simulink model "SMC_01"  (R2021a)
settings: Solver=ode14x  StartTime=0.0  StopTime=30  FixedStep=0.01  RelTol=1e-3
libraries: simulink x2
settings Model: Creator=TMP  LastModifiedBy=TMP

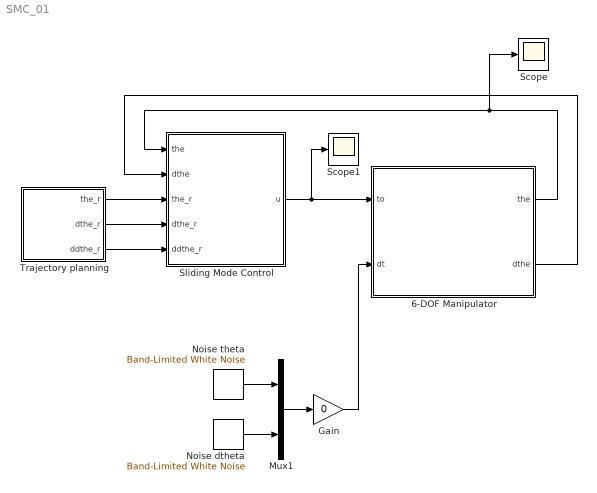
== system SMC_01 ==
  6-DOF Manipulator : Subsystem
  Gain : Gain  Gain=0
  Mux1 : Mux  Inputs=2
  Noise dtheta : simulink/Sources/Band-Limited White Noise  Cov=[0.03]  Ts=0.01  seed=[23341]
  Noise theta : simulink/Sources/Band-Limited White Noise  Cov=[0.003]  Ts=0.01  seed=[23341]
  Scope : Scope
  Scope1 : Scope
  Sliding Mode Control : MATLAB Function  TreatAsAtomicUnit=on
  Trajectory planning : Subsystem
  wires:
  Sliding Mode Control/1(u) -> Scope1/1, 6-DOF Manipulator/1(to)
  Noise theta/1 -> Mux1/1
  Noise dtheta/1 -> Mux1/2
  Gain/1 -> 6-DOF Manipulator/2(dt)
  Mux1/1 -> Gain/1
  6-DOF Manipulator/2(dthe) -> Sliding Mode Control/2(dthe)
  6-DOF Manipulator/1(the) -> Scope/1, Sliding Mode Control/1(the)
  Trajectory planning/3(ddthe_r) -> Sliding Mode Control/5(ddthe_r)
  Trajectory planning/2(dthe_r) -> Sliding Mode Control/4(dthe_r)
  Trajectory planning/1(the_r) -> Sliding Mode Control/3(the_r)

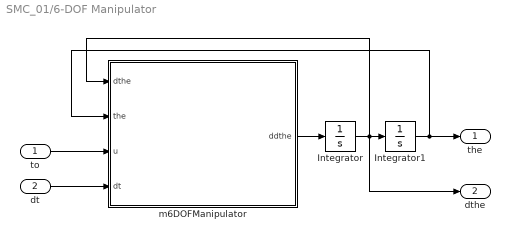
== system SMC_01/6-DOF Manipulator ==
  to : Inport
  dt : Inport  Port=2
  Integrator : Integrator  InitialCondition=[0.01;0.01;0.01;0.01;0.01;0.01]
  Integrator1 : Integrator  InitialCondition=[0.01;0.01;0.01;0.01;0.01;0.01]
  m6DOFManipulator : MATLAB Function  TreatAsAtomicUnit=on
  the : Outport
  dthe : Outport  Port=2
  wires:
  Integrator1/1 -> the/1, m6DOFManipulator/2(the)
  m6DOFManipulator/1(ddthe) -> Integrator/1
  Integrator/1 -> dthe/1, m6DOFManipulator/1(dthe), Integrator1/1
  dt/1 -> m6DOFManipulator/4(dt)
  to/1 -> m6DOFManipulator/3(u)

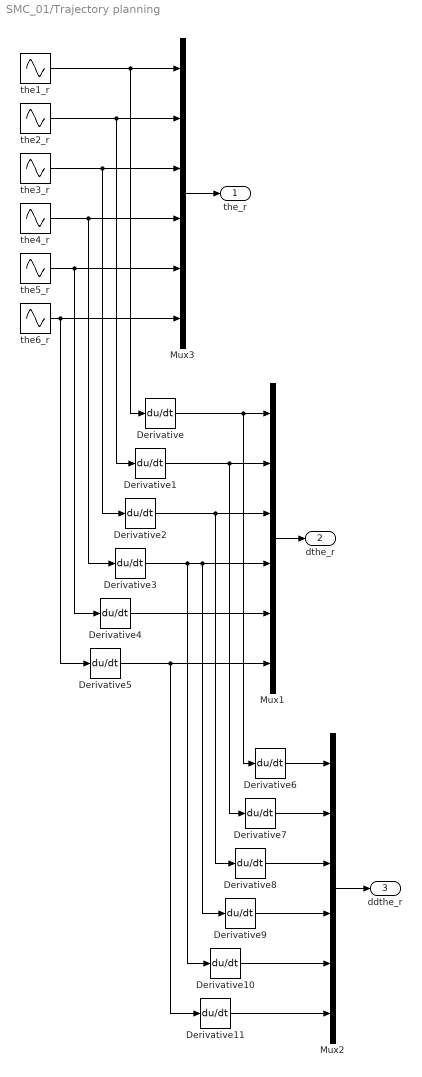
== system SMC_01/Trajectory planning ==
  Derivative{,1..11} (12 alike) : Derivative
  Mux1 : Mux  Inputs=6
  Mux2 : Mux  Inputs=6
  Mux3 : Mux  Inputs=6
  the1_r : Sin  Amplitude=pi/3  Frequency=2*pi*0.1  SampleTime=0
  the2_r : Sin  Amplitude=pi/4  Frequency=2*pi*0.1  SampleTime=0
  the3_r : Sin  Amplitude=pi/6  Frequency=2*pi*0.1  SampleTime=0
  the4_r : Sin  Amplitude=pi/3  Frequency=2*pi*0.1  Phase=pi/3  SampleTime=0
  the5_r : Sin  Amplitude=pi/4  Frequency=2*pi*0.1  Phase=pi/4  SampleTime=0
  the6_r : Sin  Amplitude=pi/6  Frequency=2*pi*0.1  Phase=pi/6  SampleTime=0
  the_r : Outport  VectorParamsAs1DForOutWhenUnconnected=off
  dthe_r : Outport  Port=2  VectorParamsAs1DForOutWhenUnconnected=off
  ddthe_r : Outport  Port=3  VectorParamsAs1DForOutWhenUnconnected=off
  wires:
  the1_r/1 -> Derivative/1, Mux3/1
  the2_r/1 -> Derivative1/1, Mux3/2
  the3_r/1 -> Derivative2/1, Mux3/3
  the4_r/1 -> Derivative3/1, Mux3/4
  the5_r/1 -> Derivative4/1, Mux3/5
  the6_r/1 -> Derivative5/1, Mux3/6
  Derivative/1 -> Derivative6/1, Mux1/1
  Derivative1/1 -> Derivative7/1, Mux1/2
  Derivative2/1 -> Derivative8/1, Mux1/3
  Derivative3/1 -> Derivative10/1, Derivative9/1, Mux1/4
  Derivative4/1 -> Mux1/5
  Derivative5/1 -> Derivative11/1, Mux1/6
  Mux3/1 -> the_r/1
  Derivative6/1 -> Mux2/1
  Derivative7/1 -> Mux2/2
  Derivative8/1 -> Mux2/3
  Derivative9/1 -> Mux2/4
  Derivative10/1 -> Mux2/5
  Derivative11/1 -> Mux2/6
  Mux1/1 -> dthe_r/1
  Mux2/1 -> ddthe_r/1

== matlab function SMC_01/Sliding Mode Control ==
  data: the input; u output; dthe input; the_r input; dthe_r input; ddthe_r input
function u = SMC(the,dthe,the_r,dthe_r,ddthe_r)
%% Declare manipulator dynamics:
m1=0.1; m2=0.1; m3=0.1; m4=0.1; m5=0.1; m6=0.1;
I1=0; I2=0; I3=0; I4=0; I5=0; I6=1;
a1=0.75; a2=2.70; a3=0.90; d1=3.35; d4=2.95; d7=0.80;
g=9.81;
%%
e1 = the(1); e2 = the(2); e3 = the(3);
e4 = the(4); e5 = the(5); e6 = the(6);
de1 = dthe(1); de2 = dthe(2); de3 = dthe(3);
de4 = dthe(4); de5 = dthe(5); de6 = dthe(6);
%% M
M = [I1 + I2 + I3 + I4 + I5 + I6 + a1^2*m2 + a1^2*m3 + a1^2*m4 + (a2^2*m3)/2 + a1^2*m5 + (a2^2*m4)/2 + a1^2*m6 + (a2^2*m5)/2 + (a3^2*m4)/2 + (a2^2*m6)/2 + (a3^2*m5)/2 + (a3^2*m6)/2 + (d4^2*m4)/2 + (d4^2*m5)/2 + (d4^2*m6)/2 - (a2^2*m3*cos(2*e2))/2 - (a2^2*m4*cos(2*e2))/2 - (a2^2*m5*cos(2*e2))/2 - (a2^2*m6*cos(2*e2))/2 - (a3^2*m4*cos(2*e2 + 2*e3))/2 - (a3^2*m5*cos(2*e2 + 2*e3))/2 - (a3^2*m6*cos(2*e2 + 2*e3))/2 + (d4^2*m4*cos(2*e2 + 2*e3))/2 + (d4^2*m5*cos(2*e2 + 2*e3))/2 + (d4^2*m6*cos(2*e2 + 2*e3))/2 + 2*a1*d4*m4*cos(e2 + e3) + 2*a1*d4*m5*cos(e2 + e3) + 2*a1*d4*m6*cos(e2 + e3) + 2*a1*a3*m4*sin(e2 + e3) + 2*a1*a3*m5*sin(e2 + e3) + 2*a1*a3*m6*sin(e2 + e3) + a2*a3*m4*cos(e3) + a2*a3*m5*cos(e3) + a2*a3*m6*cos(e3) + 2*a1*a2*m3*sin(e2) + 2*a1*a2*m4*sin(e2) + 2*a1*a2*m5*sin(e2) + 2*a1*a2*m6*sin(e2) - a2*d4*m4*sin(e3) - a2*d4*m5*sin(e3) - a2*d4*m6*sin(e3) - a2*a3*m4*cos(2*e2 + e3) - a2*a3*m5*cos(2*e2 + e3) - a2*a3*m6*cos(2*e2 + e3) + a2*d4*m4*sin(2*e2 + e3) + a2*d4*m5*sin(2*e2 + e3) + a2*d4*m6*sin(2*e2 + e3) + a3*d4*m4*sin(2*e2 + 2*e3) + a3*d4*m5*sin(2*e2 + 2*e3) + a3*d4*m6*sin(2*e2 + 2*e3),0,0,-sin(e2 + e3)*(I4 + I5 + I6),cos(e2 + e3)*sin(e4)*(I5 + I6),I6*cos(e4)*sin(e2)*sin(e3)*sin(e5) - I6*cos(e3)*cos(e5)*sin(e2) - I6*cos(e2)*cos(e3)*cos(e4)*sin(e5) - I6*cos(e2)*cos(e5)*sin(e3);
     0,I2 + I3 + I4 + I5 + I6 + a2^2*m3 + a2^2*m4 + a2^2*m5 + a3^2*m4 + a2^2*m6 + a3^2*m5 + a3^2*m6 + d4^2*m4 + d4^2*m5 + d4^2*m6 + 2*a2*a3*m4*cos(e3) + 2*a2*a3*m5*cos(e3) + 2*a2*a3*m6*cos(e3) - 2*a2*d4*m4*sin(e3) - 2*a2*d4*m5*sin(e3) - 2*a2*d4*m6*sin(e3),I3 + I4 + I5 + I6 + a3^2*m4 + a3^2*m5 + a3^2*m6 + d4^2*m4 + d4^2*m5 + d4^2*m6 + a2*a3*m4*cos(e3) + a2*a3*m5*cos(e3) + a2*a3*m6*cos(e3) - a2*d4*m4*sin(e3) - a2*d4*m5*sin(e3) - a2*d4*m6*sin(e3),0,cos(e4)*(I5 + I6),I6*sin(e4)*sin(e5);
     0,I3 + I4 + I5 + I6 + a3^2*m4 + a3^2*m5 + a3^2*m6 + d4^2*m4 + d4^2*m5 + d4^2*m6 + a2*a3*m4*cos(e3) + a2*a3*m5*cos(e3) + a2*a3*m6*cos(e3) - a2*d4*m4*sin(e3) - a2*d4*m5*sin(e3) - a2*d4*m6*sin(e3),I3 + I4 + I5 + I6 + a3^2*m4 + a3^2*m5 + a3^2*m6 + d4^2*m4 + d4^2*m5 + d4^2*m6,0,cos(e4)*(I5 + I6),I6*sin(e4)*sin(e5);
    -sin(e2 + e3)*(I4 + I5 + I6),0,0,I4 + I5 + I6,0,I6*cos(e5);
    cos(e2 + e3)*sin(e4)*(I5 + I6),cos(e4)*(I5 + I6),cos(e4)*(I5 + I6),0,I5 + I6,0;
    I6*cos(e4)*sin(e2)*sin(e3)*sin(e5) - I6*cos(e3)*cos(e5)*sin(e2) - I6*cos(e2)*cos(e3)*cos(e4)*sin(e5) - I6*cos(e2)*cos(e5)*sin(e3),I6*sin(e4)*sin(e5),I6*sin(e4)*sin(e5),I6*cos(e5),0,I6];
%% C
C = ...
[de2*(a2^2*m3*sin(2*e2) + a2^2*m4*sin(2*e2) + a2^2*m5*sin(2*e2) + a2^2*m6*sin(2*e2) + a3^2*m4*sin(2*e2 + 2*e3) + a3^2*m5*sin(2*e2 + 2*e3) + a3^2*m6*sin(2*e2 + 2*e3) - d4^2*m4*sin(2*e2 + 2*e3) - d4^2*m5*sin(2*e2 + 2*e3) - d4^2*m6*sin(2*e2 + 2*e3) + 2*a1*a3*m4*cos(e2 + e3) + 2*a1*a3*m5*cos(e2 + e3) + 2*a1*a3*m6*cos(e2 + e3) - 2*a1*d4*m4*sin(e2 + e3) - 2*a1*d4*m5*sin(e2 + e3) - 2*a1*d4*m6*sin(e2 + e3) + 2*a1*a2*m3*cos(e2) + 2*a1*a2*m4*cos(e2) + 2*a1*a2*m5*cos(e2) + 2*a1*a2*m6*cos(e2) + 2*a2*d4*m4*cos(2*e2 + e3) + 2*a2*d4*m5*cos(2*e2 + e3) + 2*a2*d4*m6*cos(2*e2 + e3) + 2*a2*a3*m4*sin(2*e2 + e3) + 2*a2*a3*m5*sin(2*e2 + e3) + 2*a2*a3*m6*sin(2*e2 + e3) + 2*a3*d4*m4*cos(2*e2 + 2*e3) + 2*a3*d4*m5*cos(2*e2 + 2*e3) + 2*a3*d4*m6*cos(2*e2 + 2*e3)) + de3*(m4 + m5 + m6)*(a3^2*sin(2*e2 + 2*e3) - d4^2*sin(2*e2 + 2*e3) + a2*d4*cos(2*e2 + e3) + a2*a3*sin(2*e2 + e3) + 2*a3*d4*cos(2*e2 + 2*e3) + 2*a1*a3*cos(e2 + e3) - 2*a1*d4*sin(e2 + e3) - a2*d4*cos(e3) - a2*a3*sin(e3)),0,0,-cos(e2 + e3)*(de2 + de3)*(I4 + I5 + I6),-(I5 + I6)*(de2*sin(e2 + e3)*sin(e4) - de4*cos(e2 + e3)*cos(e4) + de3*sin(e2 + e3)*sin(e4)),I6*de2*(cos(e5)*sin(e2)*sin(e3) - cos(e2)*cos(e3)*cos(e5) + cos(e2)*cos(e4)*sin(e3)*sin(e5) + cos(e3)*cos(e4)*sin(e2)*sin(e5)) + I6*de3*(cos(e5)*sin(e2)*sin(e3) - cos(e2)*cos(e3)*cos(e5) + cos(e2)*cos(e4)*sin(e3)*sin(e5) + cos(e3)*cos(e4)*sin(e2)*sin(e5)) + I6*de5*(cos(e2)*sin(e3)*sin(e5) + cos(e3)*sin(e2)*sin(e5) - cos(e2)*cos(e3)*cos(e4)*cos(e5) + cos(e4)*cos(e5)*sin(e2)*sin(e3)) + I6*de4*cos(e2 + e3)*sin(e4)*sin(e5);
 (I4*de4*cos(e2 + e3))/2 + (I5*de4*cos(e2 + e3))/2 + (I6*de4*cos(e2 + e3))/2 - (a2^2*de1*m3*sin(2*e2))/2 - (a2^2*de1*m4*sin(2*e2))/2 - (a2^2*de1*m5*sin(2*e2))/2 - (a2^2*de1*m6*sin(2*e2))/2 - (a3^2*de1*m4*sin(2*e2 + 2*e3))/2 - (a3^2*de1*m5*sin(2*e2 + 2*e3))/2 - (a3^2*de1*m6*sin(2*e2 + 2*e3))/2 + (d4^2*de1*m4*sin(2*e2 + 2*e3))/2 + (d4^2*de1*m5*sin(2*e2 + 2*e3))/2 + (d4^2*de1*m6*sin(2*e2 + 2*e3))/2 + (I5*de5*sin(e2 + e3)*sin(e4))/2 + (I6*de5*sin(e2 + e3)*sin(e4))/2 - a3*d4*de1*m4*cos(2*e2 + 2*e3) - a3*d4*de1*m5*cos(2*e2 + 2*e3) - a3*d4*de1*m6*cos(2*e2 + 2*e3) + (I6*de6*cos(e2)*cos(e3)*cos(e5))/2 - a1*a3*de1*m4*cos(e2 + e3) - a1*a3*de1*m5*cos(e2 + e3) - a1*a3*de1*m6*cos(e2 + e3) - (I6*de6*cos(e5)*sin(e2)*sin(e3))/2 + a1*d4*de1*m4*sin(e2 + e3) + a1*d4*de1*m5*sin(e2 + e3) + a1*d4*de1*m6*sin(e2 + e3) - a1*a2*de1*m3*cos(e2) - a1*a2*de1*m4*cos(e2) - a1*a2*de1*m5*cos(e2) - a1*a2*de1*m6*cos(e2) - a2*d4*de1*m4*cos(2*e2 + e3) - a2*d4*de1*m5*cos(2*e2 + e3) - a2*d4*de1*m6*cos(2*e2 + e3) - a2*a3*de1*m4*sin(2*e2 + e3) - a2*a3*de1*m5*sin(2*e2 + e3) - a2*a3*de1*m6*sin(2*e2 + e3) - (I6*de6*cos(e2)*cos(e4)*sin(e3)*sin(e5))/2 - (I6*de6*cos(e3)*cos(e4)*sin(e2)*sin(e5))/2,-2*a2*de3*(d4*cos(e3) + a3*sin(e3))*(m4 + m5 + m6),-a2*de3*(d4*cos(e3) + a3*sin(e3))*(m4 + m5 + m6),(de1*cos(e2 + e3)*(I4 + I5 + I6))/2,-(sin(e4)*(2*de4 - de1*sin(e2 + e3))*(I5 + I6))/2,(I6*(2*de4*cos(e4)*sin(e5) + 2*de5*cos(e5)*sin(e4) + de1*cos(e2)*cos(e3)*cos(e5) - de1*cos(e5)*sin(e2)*sin(e3) - de1*cos(e2)*cos(e4)*sin(e3)*sin(e5) - de1*cos(e3)*cos(e4)*sin(e2)*sin(e5)))/2;
 (de4*cos(e2 + e3)*(I4 + I5 + I6))/2 - (I6*de6*(cos(e5)*sin(e2)*sin(e3) - cos(e2)*cos(e3)*cos(e5) + cos(e2)*cos(e4)*sin(e3)*sin(e5) + cos(e3)*cos(e4)*sin(e2)*sin(e5)))/2 - (de1*(m4 + m5 + m6)*(a3^2*sin(2*e2 + 2*e3) - d4^2*sin(2*e2 + 2*e3) + a2*d4*cos(2*e2 + e3) + a2*a3*sin(2*e2 + e3) + 2*a3*d4*cos(2*e2 + 2*e3) + 2*a1*a3*cos(e2 + e3) - 2*a1*d4*sin(e2 + e3) - a2*d4*cos(e3) - a2*a3*sin(e3)))/2 + (de5*sin(e2 + e3)*sin(e4)*(I5 + I6))/2,(a2*(d4*cos(e3) + a3*sin(e3))*(2*de2 - de3)*(m4 + m5 + m6))/2,(a2*de2*(d4*cos(e3) + a3*sin(e3))*(m4 + m5 + m6))/2,(de1*cos(e2 + e3)*(I4 + I5 + I6))/2,-(sin(e4)*(2*de4 - de1*sin(e2 + e3))*(I5 + I6))/2,(I6*(2*de4*cos(e4)*sin(e5) + 2*de5*cos(e5)*sin(e4) + de1*cos(e2)*cos(e3)*cos(e5) - de1*cos(e5)*sin(e2)*sin(e3) - de1*cos(e2)*cos(e4)*sin(e3)*sin(e5) - de1*cos(e3)*cos(e4)*sin(e2)*sin(e5)))/2;
 - cos(e2 + e3)*(de2 + de3)*(I4 + I5 + I6) - (de5*cos(e2 + e3)*cos(e4)*(I5 + I6))/2 - (I6*de6*cos(e2 + e3)*sin(e4)*sin(e5))/2,(de5*sin(e4)*(I5 + I6))/2 - (I6*de6*cos(e4)*sin(e5))/2,(de5*sin(e4)*(I5 + I6))/2 - (I6*de6*cos(e4)*sin(e5))/2,0,((I5 + I6)*(de2*sin(e4) + de3*sin(e4) - de1*cos(e2 + e3)*cos(e4)))/2,-(I6*sin(e5)*(2*de5 + de2*cos(e4) + de3*cos(e4) + de1*cos(e2 + e3)*sin(e4)))/2;
 - (I5 + I6)*(de2*sin(e2 + e3)*sin(e4) - de4*cos(e2 + e3)*cos(e4) + de3*sin(e2 + e3)*sin(e4)) - (I6*de6*(cos(e2)*sin(e3)*sin(e5) + cos(e3)*sin(e2)*sin(e5) - cos(e2)*cos(e3)*cos(e4)*cos(e5) + cos(e4)*cos(e5)*sin(e2)*sin(e3)))/2,- de4*sin(e4)*(I5 + I6) - (I6*de6*cos(e5)*sin(e4))/2,- de4*sin(e4)*(I5 + I6) - (I6*de6*cos(e5)*sin(e4))/2,(I6*de6*sin(e5))/2,0,-(I6*(de2*cos(e5)*sin(e4) - de4*sin(e5) + de3*cos(e5)*sin(e4) + de1*cos(e2)*sin(e3)*sin(e5) + de1*cos(e3)*sin(e2)*sin(e5) + de1*cos(e4)*cos(e5)*sin(e2)*sin(e3) - de1*cos(e2)*cos(e3)*cos(e4)*cos(e5)))/2;
 I6*de2*(cos(e5)*sin(e2)*sin(e3) - cos(e2)*cos(e3)*cos(e5) + cos(e2)*cos(e4)*sin(e3)*sin(e5) + cos(e3)*cos(e4)*sin(e2)*sin(e5)) + I6*de3*(cos(e5)*sin(e2)*sin(e3) - cos(e2)*cos(e3)*cos(e5) + cos(e2)*cos(e4)*sin(e3)*sin(e5) + cos(e3)*cos(e4)*sin(e2)*sin(e5)) + I6*de5*(cos(e2)*sin(e3)*sin(e5) + cos(e3)*sin(e2)*sin(e5) - cos(e2)*cos(e3)*cos(e4)*cos(e5) + cos(e4)*cos(e5)*sin(e2)*sin(e3)) + I6*de4*cos(e2 + e3)*sin(e4)*sin(e5),I6*de4*cos(e4)*sin(e5) + I6*de5*cos(e5)*sin(e4),I6*de4*cos(e4)*sin(e5) + I6*de5*cos(e5)*sin(e4),-I6*de5*sin(e5),0,0];
%% V
V = C*dthe;
%% G
G = ...
[    
                                                                                                                                                                                              0;
g*(a2*m3*sin(e2) + a2*m4*sin(e2) + a2*m5*sin(e2) + a2*m6*sin(e2) + d4*m4*cos(e2 + e3) + d4*m5*cos(e2 + e3) + d4*m6*cos(e2 + e3) + a3*m4*sin(e2 + e3) + a3*m5*sin(e2 + e3) + a3*m6*sin(e2 + e3));
                                                                                                                                           g*(d4*cos(e2 + e3) + a3*sin(e2 + e3))*(m4 + m5 + m6);
                                                                                                                                                                                              0;
                                                                                                                                                                                              0;
                                                                                                                                                                                              0];

%% Control:
% Controler parameters
% % with noise
% lamda = 50;
% K = 30;
% K1 = 50;

% without noise
lamda = diag([20,20,20,20,20,20]);
K = diag([20,20,20,20,20,20]);
K1 = diag([5,5,5,5,5,5]);

% Designed sliding mode control
f_x = -inv(M)*V - inv(M)*G;
g_x = inv(M);
e1 = the - the_r;
e2 = dthe - dthe_r;
s = lamda*e1 + e2;
u = inv(g_x)*(-f_x + ddthe_r - lamda*e2 - K1*s - K*sign(s));
% sat
% u = inv(g_x)*(-f_x + ddthe_r - lamda*e2 - K1*s - K*min(0.1, max(-0.1, s)));

== matlab function SMC_01/6-DOF Manipulator/m6DOFManipulator ==
  data: dthe input; the input; u input; ddthe output; dt input
function ddthe  = m6DOFManipulator(dthe,the,u,dt)
%% Declare:
m1=0.1; m2=0.1; m3=0.1; m4=0.1; m5=0.1; m6=0.1;
I1=0; I2=0; I3=0; I4=0; I5=0; I6=1;
a1=0.75; a2=2.70; a3=0.90; d1=3.35; d4=2.95; d7=0.80;
g=9.81;
%%
e1 = the(1) + dt(1); e2 = the(2) + dt(1); e3 = the(3) + dt(1);
e4 = the(4) + dt(1); e5 = the(5) + dt(1); e6 = the(6) + dt(1);
de1 = dthe(1) + dt(2); de2 = dthe(2) + dt(2); de3 = dthe(3) + dt(2);
de4 = dthe(4) + dt(2); de5 = dthe(5) + dt(2); de6 = dthe(6) + dt(2);
%% M
M = [I1 + I2 + I3 + I4 + I5 + I6 + a1^2*m2 + a1^2*m3 + a1^2*m4 + (a2^2*m3)/2 + a1^2*m5 + (a2^2*m4)/2 + a1^2*m6 + (a2^2*m5)/2 + (a3^2*m4)/2 + (a2^2*m6)/2 + (a3^2*m5)/2 + (a3^2*m6)/2 + (d4^2*m4)/2 + (d4^2*m5)/2 + (d4^2*m6)/2 - (a2^2*m3*cos(2*e2))/2 - (a2^2*m4*cos(2*e2))/2 - (a2^2*m5*cos(2*e2))/2 - (a2^2*m6*cos(2*e2))/2 - (a3^2*m4*cos(2*e2 + 2*e3))/2 - (a3^2*m5*cos(2*e2 + 2*e3))/2 - (a3^2*m6*cos(2*e2 + 2*e3))/2 + (d4^2*m4*cos(2*e2 + 2*e3))/2 + (d4^2*m5*cos(2*e2 + 2*e3))/2 + (d4^2*m6*cos(2*e2 + 2*e3))/2 + 2*a1*d4*m4*cos(e2 + e3) + 2*a1*d4*m5*cos(e2 + e3) + 2*a1*d4*m6*cos(e2 + e3) + 2*a1*a3*m4*sin(e2 + e3) + 2*a1*a3*m5*sin(e2 + e3) + 2*a1*a3*m6*sin(e2 + e3) + a2*a3*m4*cos(e3) + a2*a3*m5*cos(e3) + a2*a3*m6*cos(e3) + 2*a1*a2*m3*sin(e2) + 2*a1*a2*m4*sin(e2) + 2*a1*a2*m5*sin(e2) + 2*a1*a2*m6*sin(e2) - a2*d4*m4*sin(e3) - a2*d4*m5*sin(e3) - a2*d4*m6*sin(e3) - a2*a3*m4*cos(2*e2 + e3) - a2*a3*m5*cos(2*e2 + e3) - a2*a3*m6*cos(2*e2 + e3) + a2*d4*m4*sin(2*e2 + e3) + a2*d4*m5*sin(2*e2 + e3) + a2*d4*m6*sin(2*e2 + e3) + a3*d4*m4*sin(2*e2 + 2*e3) + a3*d4*m5*sin(2*e2 + 2*e3) + a3*d4*m6*sin(2*e2 + 2*e3),0,0,-sin(e2 + e3)*(I4 + I5 + I6),cos(e2 + e3)*sin(e4)*(I5 + I6),I6*cos(e4)*sin(e2)*sin(e3)*sin(e5) - I6*cos(e3)*cos(e5)*sin(e2) - I6*cos(e2)*cos(e3)*cos(e4)*sin(e5) - I6*cos(e2)*cos(e5)*sin(e3);
     0,I2 + I3 + I4 + I5 + I6 + a2^2*m3 + a2^2*m4 + a2^2*m5 + a3^2*m4 + a2^2*m6 + a3^2*m5 + a3^2*m6 + d4^2*m4 + d4^2*m5 + d4^2*m6 + 2*a2*a3*m4*cos(e3) + 2*a2*a3*m5*cos(e3) + 2*a2*a3*m6*cos(e3) - 2*a2*d4*m4*sin(e3) - 2*a2*d4*m5*sin(e3) - 2*a2*d4*m6*sin(e3),I3 + I4 + I5 + I6 + a3^2*m4 + a3^2*m5 + a3^2*m6 + d4^2*m4 + d4^2*m5 + d4^2*m6 + a2*a3*m4*cos(e3) + a2*a3*m5*cos(e3) + a2*a3*m6*cos(e3) - a2*d4*m4*sin(e3) - a2*d4*m5*sin(e3) - a2*d4*m6*sin(e3),0,cos(e4)*(I5 + I6),I6*sin(e4)*sin(e5);
     0,I3 + I4 + I5 + I6 + a3^2*m4 + a3^2*m5 + a3^2*m6 + d4^2*m4 + d4^2*m5 + d4^2*m6 + a2*a3*m4*cos(e3) + a2*a3*m5*cos(e3) + a2*a3*m6*cos(e3) - a2*d4*m4*sin(e3) - a2*d4*m5*sin(e3) - a2*d4*m6*sin(e3),I3 + I4 + I5 + I6 + a3^2*m4 + a3^2*m5 + a3^2*m6 + d4^2*m4 + d4^2*m5 + d4^2*m6,0,cos(e4)*(I5 + I6),I6*sin(e4)*sin(e5);
    -sin(e2 + e3)*(I4 + I5 + I6),0,0,I4 + I5 + I6,0,I6*cos(e5);
    cos(e2 + e3)*sin(e4)*(I5 + I6),cos(e4)*(I5 + I6),cos(e4)*(I5 + I6),0,I5 + I6,0;
    I6*cos(e4)*sin(e2)*sin(e3)*sin(e5) - I6*cos(e3)*cos(e5)*sin(e2) - I6*cos(e2)*cos(e3)*cos(e4)*sin(e5) - I6*cos(e2)*cos(e5)*sin(e3),I6*sin(e4)*sin(e5),I6*sin(e4)*sin(e5),I6*cos(e5),0,I6];
%% C
C = ...
[de2*(a2^2*m3*sin(2*e2) + a2^2*m4*sin(2*e2) + a2^2*m5*sin(2*e2) + a2^2*m6*sin(2*e2) + a3^2*m4*sin(2*e2 + 2*e3) + a3^2*m5*sin(2*e2 + 2*e3) + a3^2*m6*sin(2*e2 + 2*e3) - d4^2*m4*sin(2*e2 + 2*e3) - d4^2*m5*sin(2*e2 + 2*e3) - d4^2*m6*sin(2*e2 + 2*e3) + 2*a1*a3*m4*cos(e2 + e3) + 2*a1*a3*m5*cos(e2 + e3) + 2*a1*a3*m6*cos(e2 + e3) - 2*a1*d4*m4*sin(e2 + e3) - 2*a1*d4*m5*sin(e2 + e3) - 2*a1*d4*m6*sin(e2 + e3) + 2*a1*a2*m3*cos(e2) + 2*a1*a2*m4*cos(e2) + 2*a1*a2*m5*cos(e2) + 2*a1*a2*m6*cos(e2) + 2*a2*d4*m4*cos(2*e2 + e3) + 2*a2*d4*m5*cos(2*e2 + e3) + 2*a2*d4*m6*cos(2*e2 + e3) + 2*a2*a3*m4*sin(2*e2 + e3) + 2*a2*a3*m5*sin(2*e2 + e3) + 2*a2*a3*m6*sin(2*e2 + e3) + 2*a3*d4*m4*cos(2*e2 + 2*e3) + 2*a3*d4*m5*cos(2*e2 + 2*e3) + 2*a3*d4*m6*cos(2*e2 + 2*e3)) + de3*(m4 + m5 + m6)*(a3^2*sin(2*e2 + 2*e3) - d4^2*sin(2*e2 + 2*e3) + a2*d4*cos(2*e2 + e3) + a2*a3*sin(2*e2 + e3) + 2*a3*d4*cos(2*e2 + 2*e3) + 2*a1*a3*cos(e2 + e3) - 2*a1*d4*sin(e2 + e3) - a2*d4*cos(e3) - a2*a3*sin(e3)),0,0,-cos(e2 + e3)*(de2 + de3)*(I4 + I5 + I6),-(I5 + I6)*(de2*sin(e2 + e3)*sin(e4) - de4*cos(e2 + e3)*cos(e4) + de3*sin(e2 + e3)*sin(e4)),I6*de2*(cos(e5)*sin(e2)*sin(e3) - cos(e2)*cos(e3)*cos(e5) + cos(e2)*cos(e4)*sin(e3)*sin(e5) + cos(e3)*cos(e4)*sin(e2)*sin(e5)) + I6*de3*(cos(e5)*sin(e2)*sin(e3) - cos(e2)*cos(e3)*cos(e5) + cos(e2)*cos(e4)*sin(e3)*sin(e5) + cos(e3)*cos(e4)*sin(e2)*sin(e5)) + I6*de5*(cos(e2)*sin(e3)*sin(e5) + cos(e3)*sin(e2)*sin(e5) - cos(e2)*cos(e3)*cos(e4)*cos(e5) + cos(e4)*cos(e5)*sin(e2)*sin(e3)) + I6*de4*cos(e2 + e3)*sin(e4)*sin(e5);
 (I4*de4*cos(e2 + e3))/2 + (I5*de4*cos(e2 + e3))/2 + (I6*de4*cos(e2 + e3))/2 - (a2^2*de1*m3*sin(2*e2))/2 - (a2^2*de1*m4*sin(2*e2))/2 - (a2^2*de1*m5*sin(2*e2))/2 - (a2^2*de1*m6*sin(2*e2))/2 - (a3^2*de1*m4*sin(2*e2 + 2*e3))/2 - (a3^2*de1*m5*sin(2*e2 + 2*e3))/2 - (a3^2*de1*m6*sin(2*e2 + 2*e3))/2 + (d4^2*de1*m4*sin(2*e2 + 2*e3))/2 + (d4^2*de1*m5*sin(2*e2 + 2*e3))/2 + (d4^2*de1*m6*sin(2*e2 + 2*e3))/2 + (I5*de5*sin(e2 + e3)*sin(e4))/2 + (I6*de5*sin(e2 + e3)*sin(e4))/2 - a3*d4*de1*m4*cos(2*e2 + 2*e3) - a3*d4*de1*m5*cos(2*e2 + 2*e3) - a3*d4*de1*m6*cos(2*e2 + 2*e3) + (I6*de6*cos(e2)*cos(e3)*cos(e5))/2 - a1*a3*de1*m4*cos(e2 + e3) - a1*a3*de1*m5*cos(e2 + e3) - a1*a3*de1*m6*cos(e2 + e3) - (I6*de6*cos(e5)*sin(e2)*sin(e3))/2 + a1*d4*de1*m4*sin(e2 + e3) + a1*d4*de1*m5*sin(e2 + e3) + a1*d4*de1*m6*sin(e2 + e3) - a1*a2*de1*m3*cos(e2) - a1*a2*de1*m4*cos(e2) - a1*a2*de1*m5*cos(e2) - a1*a2*de1*m6*cos(e2) - a2*d4*de1*m4*cos(2*e2 + e3) - a2*d4*de1*m5*cos(2*e2 + e3) - a2*d4*de1*m6*cos(2*e2 + e3) - a2*a3*de1*m4*sin(2*e2 + e3) - a2*a3*de1*m5*sin(2*e2 + e3) - a2*a3*de1*m6*sin(2*e2 + e3) - (I6*de6*cos(e2)*cos(e4)*sin(e3)*sin(e5))/2 - (I6*de6*cos(e3)*cos(e4)*sin(e2)*sin(e5))/2,-2*a2*de3*(d4*cos(e3) + a3*sin(e3))*(m4 + m5 + m6),-a2*de3*(d4*cos(e3) + a3*sin(e3))*(m4 + m5 + m6),(de1*cos(e2 + e3)*(I4 + I5 + I6))/2,-(sin(e4)*(2*de4 - de1*sin(e2 + e3))*(I5 + I6))/2,(I6*(2*de4*cos(e4)*sin(e5) + 2*de5*cos(e5)*sin(e4) + de1*cos(e2)*cos(e3)*cos(e5) - de1*cos(e5)*sin(e2)*sin(e3) - de1*cos(e2)*cos(e4)*sin(e3)*sin(e5) - de1*cos(e3)*cos(e4)*sin(e2)*sin(e5)))/2;
 (de4*cos(e2 + e3)*(I4 + I5 + I6))/2 - (I6*de6*(cos(e5)*sin(e2)*sin(e3) - cos(e2)*cos(e3)*cos(e5) + cos(e2)*cos(e4)*sin(e3)*sin(e5) + cos(e3)*cos(e4)*sin(e2)*sin(e5)))/2 - (de1*(m4 + m5 + m6)*(a3^2*sin(2*e2 + 2*e3) - d4^2*sin(2*e2 + 2*e3) + a2*d4*cos(2*e2 + e3) + a2*a3*sin(2*e2 + e3) + 2*a3*d4*cos(2*e2 + 2*e3) + 2*a1*a3*cos(e2 + e3) - 2*a1*d4*sin(e2 + e3) - a2*d4*cos(e3) - a2*a3*sin(e3)))/2 + (de5*sin(e2 + e3)*sin(e4)*(I5 + I6))/2,(a2*(d4*cos(e3) + a3*sin(e3))*(2*de2 - de3)*(m4 + m5 + m6))/2,(a2*de2*(d4*cos(e3) + a3*sin(e3))*(m4 + m5 + m6))/2,(de1*cos(e2 + e3)*(I4 + I5 + I6))/2,-(sin(e4)*(2*de4 - de1*sin(e2 + e3))*(I5 + I6))/2,(I6*(2*de4*cos(e4)*sin(e5) + 2*de5*cos(e5)*sin(e4) + de1*cos(e2)*cos(e3)*cos(e5) - de1*cos(e5)*sin(e2)*sin(e3) - de1*cos(e2)*cos(e4)*sin(e3)*sin(e5) - de1*cos(e3)*cos(e4)*sin(e2)*sin(e5)))/2;
 - cos(e2 + e3)*(de2 + de3)*(I4 + I5 + I6) - (de5*cos(e2 + e3)*cos(e4)*(I5 + I6))/2 - (I6*de6*cos(e2 + e3)*sin(e4)*sin(e5))/2,(de5*sin(e4)*(I5 + I6))/2 - (I6*de6*cos(e4)*sin(e5))/2,(de5*sin(e4)*(I5 + I6))/2 - (I6*de6*cos(e4)*sin(e5))/2,0,((I5 + I6)*(de2*sin(e4) + de3*sin(e4) - de1*cos(e2 + e3)*cos(e4)))/2,-(I6*sin(e5)*(2*de5 + de2*cos(e4) + de3*cos(e4) + de1*cos(e2 + e3)*sin(e4)))/2;
 - (I5 + I6)*(de2*sin(e2 + e3)*sin(e4) - de4*cos(e2 + e3)*cos(e4) + de3*sin(e2 + e3)*sin(e4)) - (I6*de6*(cos(e2)*sin(e3)*sin(e5) + cos(e3)*sin(e2)*sin(e5) - cos(e2)*cos(e3)*cos(e4)*cos(e5) + cos(e4)*cos(e5)*sin(e2)*sin(e3)))/2,- de4*sin(e4)*(I5 + I6) - (I6*de6*cos(e5)*sin(e4))/2,- de4*sin(e4)*(I5 + I6) - (I6*de6*cos(e5)*sin(e4))/2,(I6*de6*sin(e5))/2,0,-(I6*(de2*cos(e5)*sin(e4) - de4*sin(e5) + de3*cos(e5)*sin(e4) + de1*cos(e2)*sin(e3)*sin(e5) + de1*cos(e3)*sin(e2)*sin(e5) + de1*cos(e4)*cos(e5)*sin(e2)*sin(e3) - de1*cos(e2)*cos(e3)*cos(e4)*cos(e5)))/2;
 I6*de2*(cos(e5)*sin(e2)*sin(e3) - cos(e2)*cos(e3)*cos(e5) + cos(e2)*cos(e4)*sin(e3)*sin(e5) + cos(e3)*cos(e4)*sin(e2)*sin(e5)) + I6*de3*(cos(e5)*sin(e2)*sin(e3) - cos(e2)*cos(e3)*cos(e5) + cos(e2)*cos(e4)*sin(e3)*sin(e5) + cos(e3)*cos(e4)*sin(e2)*sin(e5)) + I6*de5*(cos(e2)*sin(e3)*sin(e5) + cos(e3)*sin(e2)*sin(e5) - cos(e2)*cos(e3)*cos(e4)*cos(e5) + cos(e4)*cos(e5)*sin(e2)*sin(e3)) + I6*de4*cos(e2 + e3)*sin(e4)*sin(e5),I6*de4*cos(e4)*sin(e5) + I6*de5*cos(e5)*sin(e4),I6*de4*cos(e4)*sin(e5) + I6*de5*cos(e5)*sin(e4),-I6*de5*sin(e5),0,0];
%% V
V = C*dthe;
%% G
G = ...
[    
                                                                                                                                                                                              0;
g*(a2*m3*sin(e2) + a2*m4*sin(e2) + a2*m5*sin(e2) + a2*m6*sin(e2) + d4*m4*cos(e2 + e3) + d4*m5*cos(e2 + e3) + d4*m6*cos(e2 + e3) + a3*m4*sin(e2 + e3) + a3*m5*sin(e2 + e3) + a3*m6*sin(e2 + e3));
                                                                                                                                           g*(d4*cos(e2 + e3) + a3*sin(e2 + e3))*(m4 + m5 + m6);
                                                                                                                                                                                              0;
                                                                                                                                                                                              0;
                                                                                                                                                                                              0];
%% 
ddthe=inv(M)*(u - C*dthe - G);
